simulink model "scalemodelsimulation"  (R2019b)
settings: Solver=ode15s  StartTime=0.0  StopTime=0.5  FixedStep=0.05  MaxStep=0.5  MinStep=0.1  RelTol=1e-2  AbsTol=1e-3
undefined symbols (not defined in the file): km
libraries: mpclib x1
settings Model: Creator=Vlad  LastModifiedBy=Vlad
settings DataIOCC: ReturnWorkspaceOutputsName=tpe2155fcc_9c3f_42dd_9b90_435354f31060

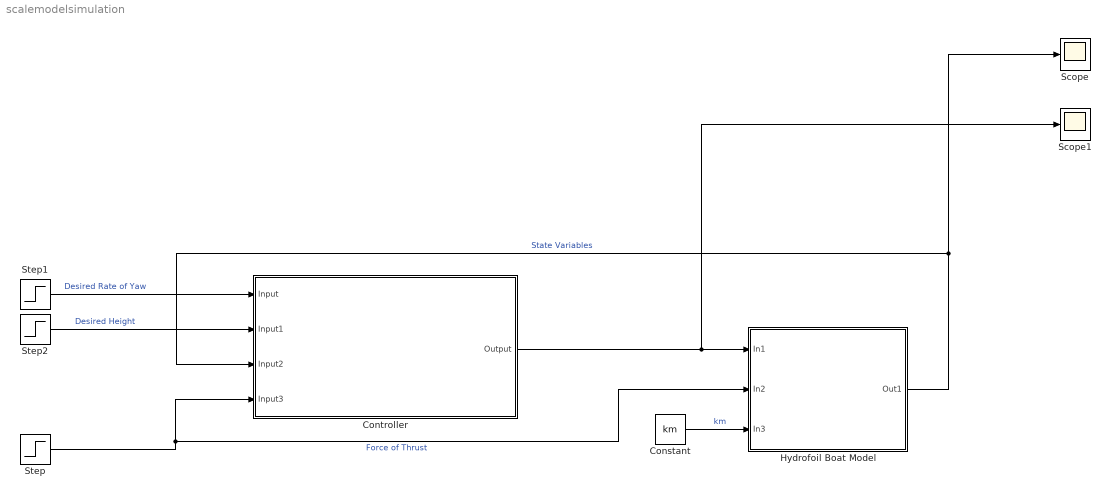
== system scalemodelsimulation ==
  Constant : Constant  Value=km
  Controller : Subsystem
  Hydrofoil Boat Model : Subsystem
  Scope : Scope
  Scope1 : Scope
  Step : Step  Time=0  After=1000  SampleTime=0
  Step1 : Step  Time=0  SampleTime=0
  Step2 : Step  Time=0  After=0  SampleTime=0
  wires:
  Controller/1(Output) -> Hydrofoil Boat Model/1(In1), Scope1/1
  Hydrofoil Boat Model/1(Out1) -> Controller/3(Input2), Scope/1  "State Variables"
  Step/1 -> Hydrofoil Boat Model/2(In2), Controller/4(Input3)  "Force of Thrust"
  Constant/1 -> Hydrofoil Boat Model/3(In3)  "km"
  Step1/1 -> Controller/1(Input)  "Desired Rate of Yaw"
  Step2/1 -> Controller/2(Input1)  "Desired Height"

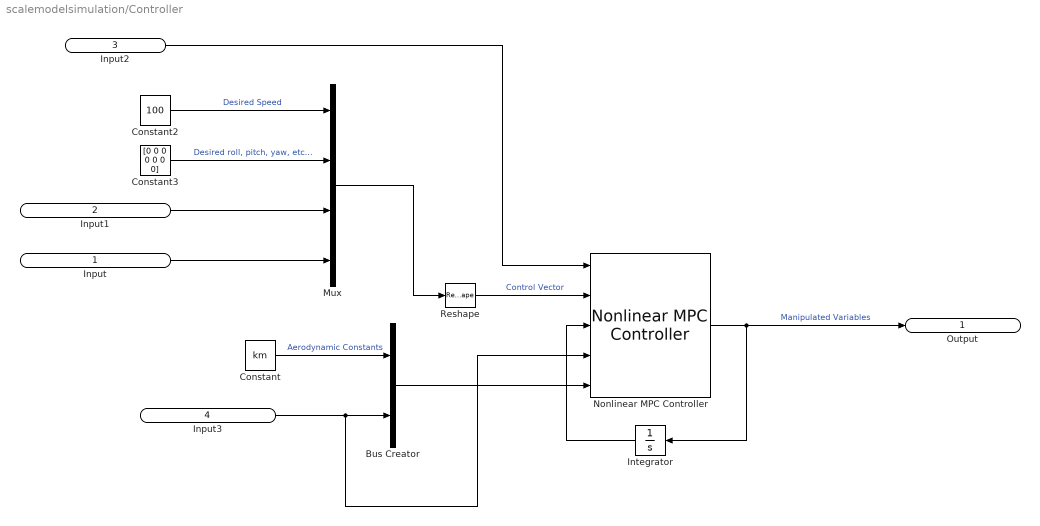
== system scalemodelsimulation/Controller ==
  Input : Inport
  Input1 : Inport  Port=2
  Input2 : Inport  Port=3
  Input3 : Inport  Port=4
  Bus Creator : BusCreator  Inputs=2  OutDataTypeStr=Bus: myBusObject_1  NonVirtualBus=on
      settings: InheritFromInputs=off
  Constant : Constant  Value=km
  Constant2 : Constant  Value=100
  Constant3 : Constant  Value=[0 0 0 0 0 0 0]
  Integrator : Integrator
  Mux : Mux
  Nonlinear MPC Controller : mpclib/Nonlinear MPC Controller  SCDEnableBlockLinearizationSpecification=on  nlmpcobj=nlobj  UseObjectTs=on  md_enabled=on  mvtarget_enabled=off  param_enabled=on  cost_enabled=off  mvseq_enabled=off  stateseq_enabled=off  ovseq_enabled=off  slack_enabled=off  status_enabled=off  ov_min=off  ov_max=off  mv_min=off  mv_max=off  mvrate_min=off  mvrate_max=off  state_min=off  state_max=off  ov_weight=off  mv_weight=off  mvrate_weight=off  ecr_weight=off  nlp_initialize=off
      settings: SourceProductName=Model Predictive Control Toolbox
  Reshape : Reshape  OutputDimensionality=Row vector (2-D)
  Output : Outport
  wires:
  Nonlinear MPC Controller/1 -> Output/1, Integrator/1  "Manipulated Variables"
  Constant3/1 -> Mux/2  "Desired roll, pitch, yaw, etc..."
  Input1/1 -> Mux/3
  Integrator/1 -> Nonlinear MPC Controller/3
  Reshape/1 -> Nonlinear MPC Controller/2  "Control Vector"
  Input3/1 -> Nonlinear MPC Controller/4, Bus Creator/2
  Input2/1 -> Nonlinear MPC Controller/1
  Input/1 -> Mux/4
  Constant2/1 -> Mux/1  "Desired Speed"
  Bus Creator/1 -> Nonlinear MPC Controller/5
  Constant/1 -> Bus Creator/1  "Aerodynamic Constants"
  Mux/1 -> Reshape/1

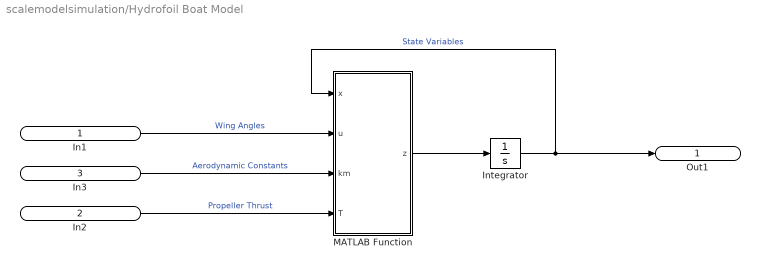
== system scalemodelsimulation/Hydrofoil Boat Model ==
  In1 : Inport
  In2 : Inport  Port=2
  In3 : Inport  Port=3
  Integrator : Integrator
  MATLAB Function : MATLAB Function  TreatAsAtomicUnit=on
  Out1 : Outport
  wires:
  Integrator/1 -> Out1/1, MATLAB Function/1(x)  "State Variables"
  In1/1 -> MATLAB Function/2(u)  "Wing Angles"
  In2/1 -> MATLAB Function/4(T)  "Propeller Thrust"
  MATLAB Function/1(z) -> Integrator/1
  In3/1 -> MATLAB Function/3(km)  "Aerodynamic Constants"

== matlab function scalemodelsimulation/Hydrofoil Boat Model/MATLAB Function ==
  data: x input; u input; km input; z output; T input
function z = fcn(x, u, km, T)
z = zeros(10,1);
z = scalemodelstatefunction(x,u,km,T);
